simulink model "adaptive_cruise_control_2019a"  (R2019a)
settings: Solver=FixedStepAuto  StartTime=0.0  StopTime=inf  RelTol=1e-3  EnableMultiTasking=on
libraries: arduinolib x5, LCDlib x1, arduinosensorlib x1
settings Model: SimulationMode=external  ExtModeTrigDuration=2  Creator=Shyam lal  LastModifiedBy=Shyam lal
settings OptimizationCC: EnhancedBackFolding=on  PassReuseOutputArgsAs=Individual arguments  MaxStackSize=64  OptimizeBlockOrder=speed  DifferentSizesBufferReuse=on  OptimizationCustomize=off
settings DebuggingCC: ParameterTunabilityLossMsg=error
settings HardwareCC: ProdBitPerInt=16  ProdBitPerPointer=16  ProdBitPerSizeT=16  ProdBitPerPtrDiffT=16  ProdLargestAtomicFloat=None  ProdWordSize=8  ProdHWDeviceType=Atmel->AVR
settings SFSimCC: MATLABDynamicMemAlloc=off
settings RTWCC: SystemTargetFile=ert.tlc  HardwareBoard=Arduino Uno  TLCOptions=-aInlineSetEventsForThisBaseRateFcn=TLC_FALSE -aSuppressMultiTaskScheduler=TLC_FALSE -aRateBasedStepFcn=1  TemplateMakefile=ert_default_tmf  GenerateReport=on  Toolchain=Arduino AVR  BuildConfiguration=Faster Runs  IncludeHyperlinkInReport=on  LaunchReport=on  GenerateTraceInfo=on  GenerateTraceReport=on  GenerateTraceReportSl=on  GenerateTraceReportSf=on  GenerateTraceReportEml=on
settings CodeAppCC: ForceParamTrailComments=on  IgnoreCustomStorageClasses=off  OperatorAnnotations=on  SimulinkDataObjDesc=on  SFDataObjDesc=on  InsertBlockDesc=on
settings ERTTargetCC: SupportContinuousTime=on  SupportVariableSizeSignals=on  ExtModeStaticAllocSize=250

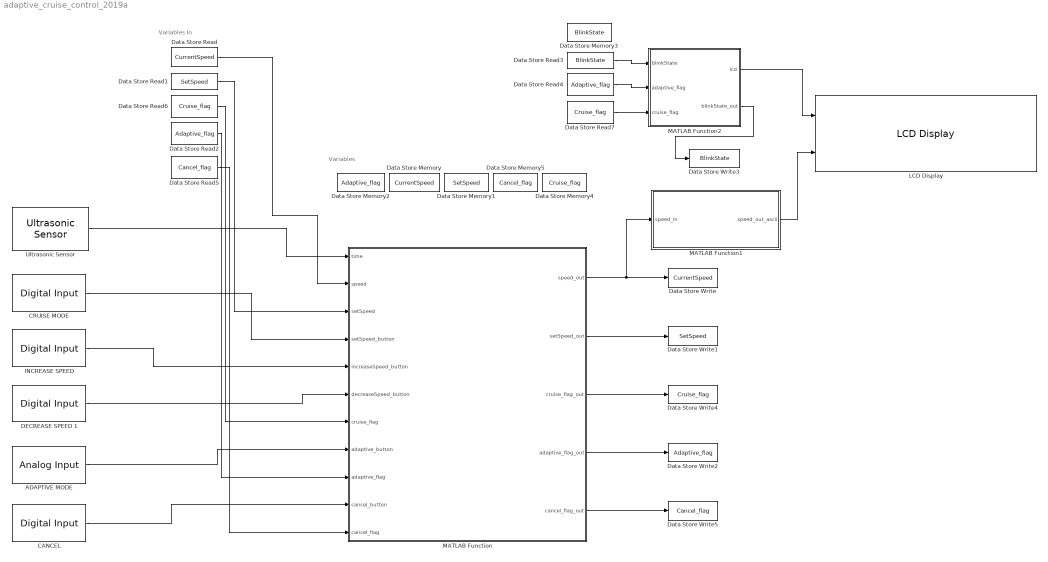
== system adaptive_cruise_control_2019a ==
  note: Variables
  note: Variables In
  ADAPTIVE MODE : arduinolib/Analog Input  pinNumber=3  ReadResultsOnly=off  ConversionTriggerSource=Software  ExternalTriggerType=uint32(0)  OutputDataType=uint16  EnableConversionCompleteNotify=off  EnableOuputStatus=off  SampleTime=.5  blockPlatform=arduino
  "CANCEL " : arduinolib/Digital Input  pinNumber=5  sampleTime=.5  blockPlatform=arduino
      settings: SourceProductName=Simulink Support Package for Arduino Hardware
  CRUISE MODE : arduinolib/Digital Input  pinNumber=4  sampleTime=.5  blockPlatform=arduino
      settings: SourceProductName=Simulink Support Package for Arduino Hardware
  DECREASE SPEED 1 : arduinolib/Digital Input  pinNumber=13  sampleTime=.5  blockPlatform=arduino
      settings: SourceProductName=Simulink Support Package for Arduino Hardware
  Data Store Memory : DataStoreMemory  DataStoreName=CurrentSpeed  ReadBeforeWriteMsg=warning  WriteAfterWriteMsg=warning  WriteAfterReadMsg=warning  ShowAdditionalParam=off
  Data Store Memory1 : DataStoreMemory  DataStoreName=SetSpeed  ReadBeforeWriteMsg=warning  WriteAfterWriteMsg=warning  WriteAfterReadMsg=warning  ShowAdditionalParam=off
  Data Store Memory2 : DataStoreMemory  DataStoreName=Adaptive_flag  ReadBeforeWriteMsg=warning  WriteAfterWriteMsg=warning  WriteAfterReadMsg=warning  ShowAdditionalParam=off
  Data Store Memory3 : DataStoreMemory  DataStoreName=BlinkState  ReadBeforeWriteMsg=warning  WriteAfterWriteMsg=warning  WriteAfterReadMsg=warning  ShowAdditionalParam=off
  Data Store Memory4 : DataStoreMemory  DataStoreName=Cruise_flag  ReadBeforeWriteMsg=warning  WriteAfterWriteMsg=warning  WriteAfterReadMsg=warning  ShowAdditionalParam=off
  Data Store Memory5 : DataStoreMemory  DataStoreName=Cancel_flag  ReadBeforeWriteMsg=warning  WriteAfterWriteMsg=warning  WriteAfterReadMsg=warning  ShowAdditionalParam=off
  Data Store Read : DataStoreRead  DataStoreName=CurrentSpeed
  Data Store Read1 : DataStoreRead  DataStoreName=SetSpeed
  Data Store Read2 : DataStoreRead  DataStoreName=Adaptive_flag
  Data Store Read3 : DataStoreRead  DataStoreName=BlinkState
  Data Store Read4 : DataStoreRead  DataStoreName=Adaptive_flag
  Data Store Read5 : DataStoreRead  DataStoreName=Cancel_flag
  Data Store Read6 : DataStoreRead  DataStoreName=Cruise_flag
  Data Store Read7 : DataStoreRead  DataStoreName=Cruise_flag
  Data Store Write : DataStoreWrite  DataStoreName=CurrentSpeed
  Data Store Write1 : DataStoreWrite  DataStoreName=SetSpeed
  Data Store Write2 : DataStoreWrite  DataStoreName=Adaptive_flag
  Data Store Write3 : DataStoreWrite  DataStoreName=BlinkState
  Data Store Write4 : DataStoreWrite  DataStoreName=Cruise_flag
  Data Store Write5 : DataStoreWrite  DataStoreName=Cancel_flag
  "INCREASE SPEED " : arduinolib/Digital Input  pinNumber=12  sampleTime=.5  blockPlatform=arduino
      settings: SourceProductName=Simulink Support Package for Arduino Hardware
  LCD Display : LCDlib/LCD Display  pins=[6,7,8,9,10,11]
      settings: SourceProductName=LCD Library
  MATLAB Function : MATLAB Function  TreatAsAtomicUnit=on
  MATLAB Function1 : MATLAB Function  TreatAsAtomicUnit=on
  MATLAB Function2 : MATLAB Function  TreatAsAtomicUnit=on
  "Ultrasonic Sensor " : arduinosensorlib/Ultrasonic Sensor  NumSignalPins=2  TrigPin=2  EchoPin=3  SignalPin=3  SampleTime_=.5  blockPlatform=ARDUINO
      settings: SourceProductName=Simulink Support Package for Arduino Hardware  SourceProductBaseCode=ARDUINO
  wires:
  MATLAB Function/1(speed_out) -> Data Store Write/1, MATLAB Function1/1(speed_in)
  MATLAB Function2/2(blinkState_out) -> Data Store Write3/1
  MATLAB Function1/1(speed_out_ascii) -> LCD Display/2
  MATLAB Function2/1(lcd) -> LCD Display/1
  Data Store Read4/1 -> MATLAB Function2/2(adaptive_flag)
  Data Store Read3/1 -> MATLAB Function2/1(blinkState)
  MATLAB Function/5(cancel_flag_out) -> Data Store Write5/1
  MATLAB Function/4(adaptive_flag_out) -> Data Store Write2/1
  MATLAB Function/3(cruise_flag_out) -> Data Store Write4/1
  MATLAB Function/2(setSpeed_out) -> Data Store Write1/1
  "CANCEL "/1 -> MATLAB Function/10(cancel_button)
  "INCREASE SPEED "/1 -> MATLAB Function/5(increaseSpeed_button)
  CRUISE MODE/1 -> MATLAB Function/4(setSpeed_button)
  DECREASE SPEED 1/1 -> MATLAB Function/6(decreaseSpeed_button)
  Data Store Read6/1 -> MATLAB Function/7(cruise_flag)
  Data Store Read2/1 -> MATLAB Function/9(adaptive_flag)
  Data Store Read/1 -> MATLAB Function/2(speed)
  Data Store Read1/1 -> MATLAB Function/3(setSpeed)
  "Ultrasonic Sensor "/1 -> MATLAB Function/1(time)
  Data Store Read5/1 -> MATLAB Function/11(cancel_flag)
  ADAPTIVE MODE/1 -> MATLAB Function/8(adaptive_button)
  Data Store Read7/1 -> MATLAB Function2/3(cruise_flag)

== matlab function adaptive_cruise_control_2019a/MATLAB Function1 ==
  data: speed_out_ascii output; speed_in input
% Program lcd_switch.m:
% Displays the current speed of the vehicle to LCD Display 
% by converting the Interger speed value to ASCII speed value using a switch case.
% Created on Feb 22, 2020 by SHYAM LAL LAKSHMIRAMIYA SRIDHAR

% Input Variables:
% speed_in = Integer value of current Speed.

% Output Variables:
% speed_out_ascii = corresponding speed value in ASCII format.

function speed_out_ascii = lcd_switch(speed_in)
switch speed_in
    case 0
        speed_out_ascii = [[48],[48]];
    case 1
        speed_out_ascii = [[48],[49]];
    case 2 
        speed_out_ascii = [[48],[50]];
    case 3
        speed_out_ascii = [[48],[51]];
    case 4
        speed_out_ascii = [[48],[52]];
    case 5
        speed_out_ascii = [[48],[53]];
    case 6
        speed_out_ascii = [[48],[54]];
    case 7
        speed_out_ascii = [[48],[55]];
    case 8
        speed_out_ascii = [[48],[56]];
    case 9
        speed_out_ascii = [[48],[57]];
    case 10
        speed_out_ascii = [[49],[48]];
    case 11 
        speed_out_ascii = [[49],[49]];
    case 12
        speed_out_ascii = [[49],[50]];
    case 13
        speed_out_ascii = [[49],[51]];
    case 14
        speed_out_ascii = [[49],[52]];
    case 15
        speed_out_ascii = [[49],[53]];
    case 16
        speed_out_ascii = [[49],[54]];
    case 17
        speed_out_ascii = [[49],[55]];
    case 18
        speed_out_ascii = [[49],[56]];
    case 19
        speed_out_ascii = [[49],[57]];
    case 20
        speed_out_ascii = [[50],[48]];
    case 21 
        speed_out_ascii = [[50],[49]];
    case 22
        speed_out_ascii = [[50],[50]];
    case 23
        speed_out_ascii = [[50],[51]];
    case 24
        speed_out_ascii = [[50],[52]];
    case 25
        speed_out_ascii = [[50],[53]];
    case 26
        speed_out_ascii = [[50],[54]];
    case 27
        speed_out_ascii = [[50],[55]];
    case 28
        speed_out_ascii = [[50],[56]];
    case 29
        speed_out_ascii = [[50],[57]];
    case 30
        speed_out_ascii = [[51],[48]];
    case 31 
        speed_out_ascii = [[51],[49]];
    case 32
        speed_out_ascii = [[51],[50]];
    case 33
        speed_out_ascii = [[51],[51]];
    case 34
        speed_out_ascii = [[51],[52]];
    case 35
        speed_out_ascii = [[51],[53]];
    case 36
        speed_out_ascii = [[51],[54]];
    case 37
        speed_out_ascii = [[51],[55]];
    case 38
        speed_out_ascii = [[51],[56]];
    case 39
        speed_out_ascii = [[51],[57]];
    case 40
        speed_out_ascii = [[52],[48]];
    case 41 
        speed_out_ascii = [[52],[49]];
    case 42
        speed_out_ascii = [[52],[50]];
    case 43
        speed_out_ascii = [[52],[51]];
    case 44
        speed_out_ascii = [[52],[52]];
    case 45
        speed_out_ascii = [[52],[53]];
    case 46
        speed_out_ascii = [[52],[54]];
    case 47
        speed_out_ascii = [[52],[55]];
    case 48
        speed_out_ascii = [[52],[56]];
    case 49
        speed_out_ascii = [[52],[57]];
    case 50
        speed_out_ascii = [[53],[48]];
    case 51 
        speed_out_ascii = [[53],[49]];
    case 52
        speed_out_ascii = [[53],[50]];
    case 53
        speed_out_ascii = [[53],[51]];
    case 54
        speed_out_ascii = [[53],[52]];
    case 55
        speed_out_ascii = [[53],[53]];
    case 56
        speed_out_ascii = [[53],[54]];
    case 57
        speed_out_ascii = [[53],[55]];
    case 58
        speed_out_ascii = [[53],[56]];
    case 59
        speed_out_ascii = [[53],[57]];
    case 60
        speed_out_ascii = [[54],[48]];
    case 61 
        speed_out_ascii = [[54],[49]];
    case 62
        speed_out_ascii = [[54],[50]];
    case 63
        speed_out_ascii = [[54],[51]];
    case 64
        speed_out_ascii = [[54],[52]];
    case 65
        speed_out_ascii = [[54],[53]];
    case 66
        speed_out_ascii = [[54],[54]];
    case 67
        speed_out_ascii = [[54],[55]];
    case 68
        speed_out_ascii = [[54],[56]];
    case 69
        speed_out_ascii = [[54],[57]];
    case 70
        speed_out_ascii = [[55],[48]];
    case 71 
        speed_out_ascii = [[55],[49]];
    case 72
        speed_out_ascii = [[55],[50]];
    case 73
        speed_out_ascii = [[55],[51]];
    case 74
        speed_out_ascii = [[55],[52]];
    case 75
        speed_out_ascii = [[55],[53]];
    case 76
        speed_out_ascii = [[55],[54]];
    case 77
        speed_out_ascii = [[55],[55]];
    case 78
        speed_out_ascii = [[55],[56]];
    case 79
        speed_out_ascii = [[55],[57]];
    case 80
        speed_out_ascii = [[56],[48]];
    case 81 
        speed_out_ascii = [[56],[49]];
    case 82
        speed_out_ascii = [[56],[50]];
    case 83
        speed_out_ascii = [[56],[51]];
    case 84
        speed_out_ascii = [[56],[52]];
    case 85
        speed_out_ascii = [[56],[53]];
    case 86
        speed_out_ascii = [[56],[54]];
    case 87
        speed_out_ascii = [[56],[55]];
    case 88
        speed_out_ascii = [[56],[56]];
    case 89
        speed_out_ascii = [[56],[57]];
    case 90
        speed_out_ascii = [[57],[48]];
    case 91 
        speed_out_ascii = [[57],[49]];
    case 92
        speed_out_ascii = [[57],[50]];
    case 93
        speed_out_ascii = [[57],[51]];
    case 94
        speed_out_ascii = [[57],[52]];
    case 95
        speed_out_ascii = [[57],[53]];
    case 96
        speed_out_ascii = [[57],[54]];
    case 97
        speed_out_ascii = [[57],[55]];
    case 98
        speed_out_ascii = [[57],[56]];
    case 99
        speed_out_ascii = [[57],[57]];
    otherwise
        speed_out_ascii = [[48],[48]];
end

== matlab function adaptive_cruise_control_2019a/MATLAB Function ==
  data: time input; speed_out output; speed input; setSpeed input; setSpeed_button input; increaseSpeed_button input; decreaseSpeed_button input; cruise_flag input; setSpeed_out output; cruise_flag_out output; adaptive_button input; adaptive_flag input; adaptive_flag_out output; cancel_button input; cancel_flag input; cancel_flag_out output
% Program Adaptive_Cruise_Control.m:
% Adjusts the speed of a car based on the obstacle in front along with
% normal cruise mode(maintaining a constant speed)
% Created on Feb 22, 2020 by SHYAM LAL LAKSHMIRAMIYA SRIDHAR

% Input Variables:
% time = time taken for the ultrasonic waves to reach the receiver end of
% the ultrasonic sensor.
% speed = current speed of the vehicle.
% setSpeed = locked speed of the vehicle in cruise mode.
% setSpeed_button = input from cruise mode button.
% increaseSpeed_button = input from increase speed button.
% decreaseSpeed_button = input from decrease speed button.
% cruise_flag = flag to represent the vehicle in cruise mode.
% adaptive_button = input from the adaptive cruise button.
% adaptive_flag = flag to represent the vehicle in Adaptive Cruise mode.
% cancel_button = input from the cancel mode button
% cancel_flag = flag to represent the vehicle is not in any driving mode.

% Output Variables:
% speed_out = updated current speed of the vehicle.
% setSpeed_out = updated locked speed of the vehicle in cruise mode. 
% cruise_flag_out = updated flag to represent the vehicle in cruise mode.
% adaptive_flag_out = updated flag to represent the vehicle in Adaptive Cruise mode.
% cancel_flag_out = updated flag to represent the vehicle is not in any driving mode.

function [speed_out, setSpeed_out,cruise_flag_out, adaptive_flag_out, cancel_flag_out] = Adaptive_Cruise_Control(time,speed,setSpeed,setSpeed_button,increaseSpeed_button, decreaseSpeed_button,cruise_flag,adaptive_button,adaptive_flag,cancel_button,cancel_flag)
    % Calculating the distance of the obstacle in front of the ultrasonic sensor.
    % Speed of sound(in air) = 343 m/s.
    % time = time for the ultrasonic waves to travel from transmitter to
    % obstacle and back to the receiver of the ultrasonic sensor.
    distance=(time*343)/2; 
    
    % Setting flags for different driving modes.
    if cancel_button % Checking cancel button input and resetting all other modes flags.
        cancel_flag_out=1;
        adaptive_flag_out=0;
        setSpeed_out=setSpeed;
        cruise_flag_out=0;
    elseif adaptive_button>600 % Checking adaptive button input and setting the adaptive cruise mode flags.
        setSpeed_out=speed;
        adaptive_flag_out=1;
        cancel_flag_out=0;
        cruise_flag_out=0;
    elseif setSpeed_button % Checking set button input and setting the normal cruise mode flags.
        setSpeed_out=speed; % Locking the current speed
        cruise_flag_out=1;
        cancel_flag_out=cancel_flag;
        adaptive_flag_out=0;
    else % Retaining flag values when not in any mode.
        setSpeed_out=setSpeed;
        cruise_flag_out=cruise_flag;
        adaptive_flag_out=adaptive_flag;
        cancel_flag_out=cancel_flag;
    end
    
    if increaseSpeed_button && ~adaptive_flag
        speed_out = speed+1; % Increasing Speed 
    elseif decreaseSpeed_button && speed>0 && ~adaptive_flag
        speed_out = speed-1; % Decreasing Speed 
    elseif cruise_flag % Cruise Mode
        if increaseSpeed_button && ~adaptive_flag % increase speed and lock.
            speed_out = speed+1;
            setSpeed_out = speed_out;
        elseif decreaseSpeed_button && speed>0 && ~adaptive_flag % decrease speed and lock.
            speed_out = speed-1;
            setSpeed_out = speed_out;
        else
            speed_out = speed;
            setSpeed_out = speed_out;
        end
    elseif adaptive_flag % Adaptive Cruise Mode
        if (distance<20) && (speed>0)
            speed_out=speed-2; % Decreasing speed by 2 if the obstacle is very near to the car.
        elseif (distance>=20) && (distance<30) && (speed>0)
            speed_out=speed-1; % Decreasing speed by 1 if the obstacle is near to the car.
        else % Bringing the speed to the set speed if no obstacle is found.
            if setSpeed==0
                speed_out=speed;
            else
                if speed<setSpeed
                    if distance<=30
                        speed_out=speed;
                    else
                        speed_out=speed+1;
                    end
                elseif speed>setSpeed && speed>0
                    speed_out=speed-1;
                else
                    speed_out=speed;
                end
            end
        end
    elseif cancel_flag || cancel_flag_out % Bring the current speed to 0.
        if speed>0
            speed_out=speed-1;
        else
            speed_out=speed;
            cancel_flag_out=0;
        end
    else % Bring the current speed to 0 if not in any mode.
        if speed>0
            speed_out=speed-1;
        else
            speed_out=speed;
        end
    end
end

== matlab function adaptive_cruise_control_2019a/MATLAB Function2 ==
  data: lcd output; blinkState input; blinkState_out output; adaptive_flag input; cruise_flag input
% Program blinkFcn.m:
% Blink the LCD Display for differentiating ACC Mode.
% Created on Feb 22, 2020 by SHYAM LAL LAKSHMIRAMIYA SRIDHAR

% Input Variables:
% blinkState = flag to represent the blinking toggle value.
% adaptive_flag = flag to represent the vehicle in Adaptive Cruise mode.

% Output Variables:
% lcd = input to the Line 2 of LCD Display.
% blinkState_out = update flag to represent the blinking toggle value.
function [lcd,blinkState_out]  = blinkFcn(blinkState,adaptive_flag,cruise_flag)

    if blinkState==0 && adaptive_flag % display blank screen in ACC mode.
        lcd=[[32],[32],[32],[32],[32],[32],[32],[32],[32],[32],[32],[32],[32]];
        blinkState_out=1;
    elseif blinkState==1 && adaptive_flag % display current speed in ACC mode.
        lcd=[[65],[67],[67],[32],[83],[112],[101],[101],[100],[58],[32],[32],[32]]; 
        blinkState_out=0;
    elseif cruise_flag % display current speed in Cruise Control mode.
        lcd=[[67],[114],[117],[105],[115],[101],[32],[83],[112],[101],[101],[100],[58]];
        blinkState_out=blinkState;
    else % display current speed in other modes/ no mode.
        lcd=[[83],[112],[101],[101],[100],[58],[32],[32],[32],[32],[32],[32],[32]];
        blinkState_out=blinkState;
    end
end
